simulink model "citt_generated_model"  (R2026b)
settings: Solver=ode15s  StopTime=citt_stop_time_s  MaxStep=1e-4  RelTol=1e-4
model workspace (MAT data in the model file):
  A_clamp_gain = 10
  C_LP = 1e-07
  C_LP_ALT = 0.0001
  F_ADC = 500
  F_ECG = 5
  F_INT = 60
  R_LP = 39800
  T_ADC = 0.002
  V_ECG_amp = 0.001
  V_INT_amp = Simulink.Parameter
  V_INT_amp.Value = 0.001
  V_INT_amp.Complexity = 'real'
  V_INT_amp.Dimensions = [1 1]
  V_INT_amp.Description = 'Placeholder default for unspecified 60 Hz interference amplitude; block keeps symbolic parameter V_INT_amp for CiTT/user tuning.'
  citt_Cf_F = 1e-08
  citt_Rf_ohm = 1000000
  citt_Vref_V = 0
  citt_adc_bits = 12
  citt_adc_vref_hi_V = 3.3
  citt_adc_vref_lo_V = 0
  citt_bioavailability = 1
  citt_ka_per_s = 0.02
  citt_ke_per_s = 0.002
  citt_opamp_input_resistance_ohm = 1000000000
  citt_opamp_open_loop_gain = 100000
  citt_opamp_output_offset_V = 0
  citt_opamp_output_resistance_ohm = 10
  citt_opamp_pole_frequency_Hz = 100000
  citt_pk_scale_uM = 10
  citt_sensor_sensitivity_A_per_uM = 2.5e-08
  citt_stop_time_s = 200
  citt_tau_m_s = 4
  citt_vminus_V = 0
  citt_vplus_V = 3.3
  model_note_V_INT_amp = 'V_INT_amp was unspecified in the source spec; it is a named tunable parameter with a placeholder default, not source authority.'
  t_step = 0.01
  t_stop = 0.1
libraries: fl_lib x5, nesl_utility x4, ee_lib x3
settings Model: Creator=Raalm  LastModifiedBy=Raalm
settings SimscapeCC: SimscapeLogType=all  SimscapeNominalValues="[{\"value\":\"1\",\"unit\":\"A\"},{\"value\":\"1\",\"unit\":\"bar\"},{\"value\":\"1\",\"unit\":\"cm^2\"},{\"value\":\"1\",\"unit\":\"cm^3/s\"},{\"value\":\"1\",\"unit\":\"kJ/kg\"},{\"value\":\"1\",\"unit\":\"kW\"},{\"value\":\"1\",\"unit\":\"l\"},{\"value\":\"1\",\"unit\":\"N\"},{\"value\":\"1\",\"unit\":\"N*m\"},{\"value\":\"1\",\"unit\":\"V\"},{\"value\":\"0.001\",\"unit\":\"Wb\"}]"  SimscapeUseEnergyAccounting=off

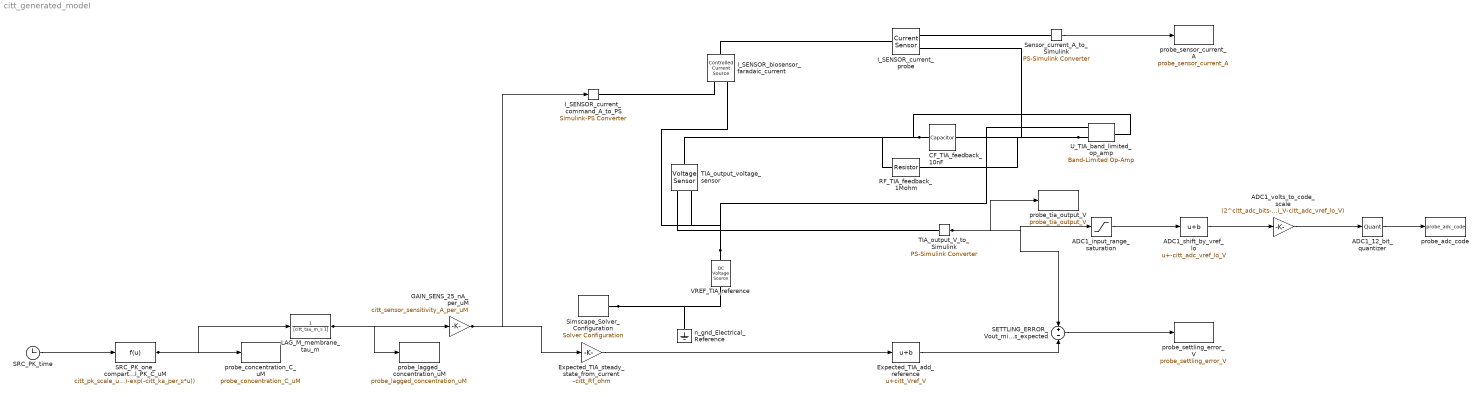
== system citt_generated_model ==
  ADC1_12_bit_quantizer : Quantizer  QuantizationInterval=1
  ADC1_input_range_saturation : Saturate  UpperLimit=citt_adc_vref_hi_V  LowerLimit=citt_adc_vref_lo_V
  ADC1_shift_by_vref_lo : Bias  Bias=-citt_adc_vref_lo_V
  ADC1_volts_to_code_scale : Gain  Gain=(2^citt_adc_bits-1)/(citt_adc_vref_hi_V-citt_adc_vref_lo_V)
  CF_TIA_feedback_10nF : ee_lib/Passive/Capacitor  cap_option=ee.enum.passive.capacitor.capOption.const  c=citt_Cf_F F  Cvec=[1e-05, 1e-06] F  Vvec=[0, 10] V  CV_table_symmetry=ee.enum.passive.capacitor.tableSymmetry.yes  f_vec=[1, 10] kHz  DFext_vec=[.8, 1.2]  enable_C_tol=ee.enum.toleranceApplication.none  averaging_period=0 s  C_tol=5  tol_distribution=ee.enum.toleranceDistribution.uniform  nSigma=4  r=0 Ohm  g=0 1/Ohm  enable_operating_limits=ee.enum.enable.no  operating_limit_action=ee.enum.passive.reportOpLim.warn  max_working_voltage_range=[-25, 25] V  power_rating=1 W  maxTemperature=85 degC  thermalEnable=false  thermalMass=1 J/K  i_specify=off  i_priority=None  i=0 A  i_nominal_specify=off  i_nominal_value=1  i_nominal_unit=A  v_specify=off  v_priority=None  v=0 V  v_nominal_specify=off  v_nominal_value=1  v_nominal_unit=V  vc_specify=off  vc_priority=High  vc=0 V  vc_nominal_specify=off  vc_nominal_value=1  vc_nominal_unit=V  T_specify=off  T_priority=None  T=298.15 K  T_nominal_specify=off  T_nominal_value=1  T_nominal_unit=K
  Expected_TIA_add_reference : Bias  Bias=citt_Vref_V
  Expected_TIA_steady_state_from_current : Gain  Gain=-citt_Rf_ohm
  GAIN_SENS_25_nA_per_uM : Gain  Gain=citt_sensor_sensitivity_A_per_uM
  I_SENSOR_biosensor_faradaic_current : fl_lib/Electrical/Electrical Sources/Controlled Current Source
  I_SENSOR_current_command_A_to_PS : nesl_utility/Simulink-PS Converter  PhysicalDomain=network_engine_domain  SubClassName=ps_input  LeftPortType=input  RightPortType=output  PseudoPeriodic=off  Frequencies=[]  NoiseDistribution=none  NoiseParameters=[]  Unit=A  AffineConversion=off  FilteringAndDerivatives=provide  SimscapeFilterOrder=1  InputFilterTimeConstant=0.001  UdotUserProvided=0
  I_SENSOR_current_probe : fl_lib/Electrical/Electrical Sensors/Current Sensor
  LAG_M_membrane_tau_m : TransferFcn  Denominator=[citt_tau_m_s 1]
  RF_TIA_feedback_1Mohm : ee_lib/Passive/Resistor  R=citt_Rf_ohm Ohm  enable_R_tol=ee.enum.toleranceApplication.none  R_tol=5  tol_distribution=ee.enum.toleranceDistribution.uniform  nSigma=4  enable_operating_limits=ee.enum.enable.no  operating_limit_action=ee.enum.passive.reportOpLim.warn  power_rating=1 W  max_working_voltage=100 V  noise_mode=ee.enum.sources.noise.Disabled  Tdevice=25 degC  sample_time=1e-3 s  repeatability=ee.enum.ic.repeatability.notRepeatable  user_seed=0  auto_seed=3911201636  power_derating_T1=70 degC  power_derating_T2=155 degC  operating_temperature_range_vec=[-50, 150] degC  alpha=3.93e-3 1/K  Tmeas=25 degC  thermal_mass=100 J/K  temperature_specify=off  temperature_priority=High  temperature=298.15 K  temperature_nominal_specify=off  temperature_nominal_value=1  temperature_nominal_unit=K
  SETTLING_ERROR_Vout_minus_expected : Sum  Inputs=+-
  SRC_PK_one_compartment_oral_PK_C_uM : Fcn  Expr=citt_pk_scale_uM*citt_bioavailability*citt_ka_per_s/(citt_ka_per_s-citt_ke_per_s)*(exp(-citt_ke_per_s*u)-exp(-citt_ka_per_s*u))
  SRC_PK_time : Clock
  Sensor_current_A_to_Simulink : nesl_utility/PS-Simulink Converter  PhysicalDomain=network_engine_domain  SubClassName=ps_output  LeftPortType=input  RightPortType=output  PseudoPeriodic=off  Frequencies=[]  VectorFormat=inherit  Unit=A  AffineConversion=off
  Simscape_Solver_Configuration : nesl_utility/Solver Configuration  PhysicalDomain=network_engine_domain  SubClassName=solver  LeftPortType=input  RightPortType=generic  Tones=[]  Harmonics=[]  SimulateNoise=off  Profile=off  UseLocalSampling=off  EnableSwitchedLinearOptims=on  FrequencyDomain=off  UseCCode=off  RelTol=0.001  AbsTol=0.001  MinStep=1e-09  ToWorkspace=off  RevertToSquareIcSolve=off  NumHomotopyIterations=100  PhasorMode=off  PhasorModeNumHarmonics=1  ConsistencySolver=NEWTON_XTOL_AFTER_FTOL  CanonicalOrdering=CANONICAL  OptimizeIntermediates=OPTIMIZED  MulticoreSolverChoice=BACKWARD_EULER  IndexReductionMethod=DerivativeReplacement  DoDC=off  ResidualTolerance=1e-09  ConsistencyTolSource=GLOBAL  ConsistencyAbsTol=0.001  ConsistencyRelTol=0.001  ConsistencyTolFactor=0.001  UseLocalSolver=off  LocalSolverChoice=NE_BACKWARD_EULER_ADVANCER  ResolveIndetEquations=on  FunctionEvalNumThread=1  LocalSolverSampleTime=0.001  DoFixedCost=off  MaxNonlinIter=3  MaxModeIter=2  ComputeImpulses=off  ImpulseIterations=2  LinearAlgebra=auto  LinearAlgebraNumThread=0  EquationFormulation=NE_TIME_EF  DelaysMemoryBudget=1024  AutomaticFiltering=on  FilteringTimeConstant=0.001  PartitionStorageMethod=AS_NEEDED  PartitionMemoryBudget=1024  PartitionMethod=BALANCED  MultibodyUseLocalSolver=off  MultibodyLocalSolverChoice=ODE1  MultibodyLocalSolverSampleTime=0.001
  TIA_output_V_to_Simulink : nesl_utility/PS-Simulink Converter  PhysicalDomain=network_engine_domain  SubClassName=ps_output  LeftPortType=input  RightPortType=output  PseudoPeriodic=off  Frequencies=[]  VectorFormat=inherit  Unit=V  AffineConversion=off
  TIA_output_voltage_sensor : fl_lib/Electrical/Electrical Sensors/Voltage Sensor
  U_TIA_band_limited_op_amp : ee_lib/Integrated Circuits/Band-Limited Op-Amp  A=citt_opamp_open_loop_gain  Rin=citt_opamp_input_resistance_ohm Ohm  Rout=citt_opamp_output_resistance_ohm Ohm  Vmin=citt_vminus_V V  Vmax=citt_vplus_V V  Vdotmax=1000 V/s  f=citt_opamp_pole_frequency_Hz Hz  V0=citt_opamp_output_offset_V V
  VREF_TIA_reference : fl_lib/Electrical/Electrical Sources/DC Voltage Source  v0=citt_Vref_V V
  n_gnd_Electrical_Reference : fl_lib/Electrical/Electrical Elements/Electrical Reference
  probe_adc_code : ToWorkspace  VariableName=probe_adc_code  SaveFormat=Structure With Time  SampleTime=-1
  probe_concentration_C_uM : ToWorkspace  VariableName=probe_concentration_C_uM  SaveFormat=Structure With Time  SampleTime=-1
  probe_lagged_concentration_uM : ToWorkspace  VariableName=probe_lagged_concentration_uM  SaveFormat=Structure With Time  SampleTime=-1
  probe_sensor_current_A : ToWorkspace  VariableName=probe_sensor_current_A  SaveFormat=Structure With Time  SampleTime=-1
  probe_settling_error_V : ToWorkspace  VariableName=probe_settling_error_V  SaveFormat=Structure With Time  SampleTime=-1
  probe_tia_output_V : ToWorkspace  VariableName=probe_tia_output_V  SaveFormat=Structure With Time  SampleTime=-1
  wires:
  SRC_PK_time/1 -> SRC_PK_one_compartment_oral_PK_C_uM/1
  SRC_PK_one_compartment_oral_PK_C_uM/1 -> probe_concentration_C_uM/1, LAG_M_membrane_tau_m/1
  LAG_M_membrane_tau_m/1 -> probe_lagged_concentration_uM/1, GAIN_SENS_25_nA_per_uM/1
  GAIN_SENS_25_nA_per_uM/1 -> Expected_TIA_steady_state_from_current/1, I_SENSOR_current_command_A_to_PS/1
  Sensor_current_A_to_Simulink/1 -> probe_sensor_current_A/1
  TIA_output_V_to_Simulink/1 -> probe_tia_output_V/1, ADC1_input_range_saturation/1, SETTLING_ERROR_Vout_minus_expected/1
  ADC1_input_range_saturation/1 -> ADC1_shift_by_vref_lo/1
  ADC1_shift_by_vref_lo/1 -> ADC1_volts_to_code_scale/1
  ADC1_volts_to_code_scale/1 -> ADC1_12_bit_quantizer/1
  ADC1_12_bit_quantizer/1 -> probe_adc_code/1
  Expected_TIA_steady_state_from_current/1 -> Expected_TIA_add_reference/1
  Expected_TIA_add_reference/1 -> SETTLING_ERROR_Vout_minus_expected/2
  SETTLING_ERROR_Vout_minus_expected/1 -> probe_settling_error_V/1
  connections:
  I_SENSOR_current_command_A_to_PS/RConn1 -- I_SENSOR_biosensor_faradaic_current/RConn1
  I_SENSOR_biosensor_faradaic_current/LConn1 -- I_SENSOR_current_probe/LConn1
  U_TIA_band_limited_op_amp/LConn2 -- CF_TIA_feedback_10nF/RConn1 -- I_SENSOR_current_probe/RConn2 -- RF_TIA_feedback_1Mohm/RConn1
  VREF_TIA_reference/LConn1 -- TIA_output_voltage_sensor/RConn2 -- I_SENSOR_biosensor_faradaic_current/RConn2 -- U_TIA_band_limited_op_amp/LConn1
  n_gnd_Electrical_Reference/LConn1 -- Simscape_Solver_Configuration/RConn1 -- VREF_TIA_reference/RConn1
  U_TIA_band_limited_op_amp/RConn1 -- TIA_output_voltage_sensor/LConn1 -- CF_TIA_feedback_10nF/LConn1 -- RF_TIA_feedback_1Mohm/LConn1
  TIA_output_voltage_sensor/RConn1 -- TIA_output_V_to_Simulink/LConn1
  I_SENSOR_current_probe/RConn1 -- Sensor_current_A_to_Simulink/LConn1
